simulink model "Ej1_sim"  (R2021a)
settings: Solver=VariableStepAuto  StartTime=0.0  StopTime=5  RelTol=1e-3
libraries: cstblocks x2
settings Model: Creator=crist  LastModifiedBy=crist

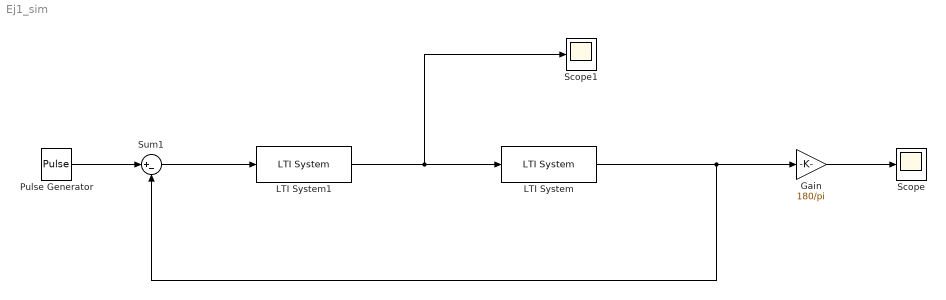
== system Ej1_sim ==
  Gain : Gain  Gain=180/pi
  LTI System : cstblocks/LTI System  sys=P  IC=[]
  LTI System1 : cstblocks/LTI System  sys=C  IC=[]
  Pulse Generator : DiscretePulseGenerator  PulseType=Time based  Amplitude=5*pi/180  Period=10  PulseWidth=0.5
  Scope : Scope
  Scope1 : Scope
  Sum1 : Sum  Inputs=|+-
  wires:
  Pulse Generator/1 -> Sum1/1
  LTI System/1 -> Sum1/2, Gain/1
  LTI System1/1 -> Scope1/1, LTI System/1
  Sum1/1 -> LTI System1/1
  Gain/1 -> Scope/1
